simulink model "test_motor_model"  (Simulink 7.1)
settings: Solver=ode113  StartTime=0.0  StopTime=0.3  RelTol=1e-3
undefined symbols (not defined in the file or in its folder): Cog_sm, J_sm, Km_sm, L_sm, P0_sm, R_sm, Sm_sm
settings Model: Creator=dep06435  LastModifiedBy=dep06435  ExtModeTrigMode=oneshot  ExtModeArmWhenConnect=off
settings DataIOCC: LimitDataPoints=off  SaveOutput=off  SaveTime=off
settings OptimizationCC: BlockReduction=off  BooleanDataType=off
settings DebuggingCC: SaveWithParameterizedLinksMsg=none  SignalResolutionControl=TryResolveAllWithWarning  SolverPrmCheckMsg=none  MultiTaskDSMMsg=warning  MultiTaskCondExecSysMsg=none  StrictBusMsg=None
settings HardwareCC: TargetUnknown=on
settings RTWCC: IncludeERTFirstTime=on
settings STFCustomTargetCC: ModelReferenceCompliant=off  SystemTargetFile=grt.tlc

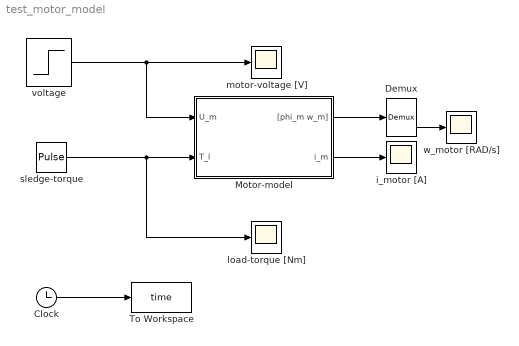
== system test_motor_model ==
  Clock : Clock
      settings: Decimation=10
  Demux : Demux  Outputs=2
  Motor-model : Subsystem  mask(Motor-model 1 VVR-41-AH-98004){km=Km_sm, Rm=R_sm, Jm=J_sm, Lm=L_sm, Sm=Sm_sm, Fc=Cog_sm, phim0=P0_sm}
      mask prompts: km "Motor-constant km [Nm/A]"; Rm "Motor-resistance R [ohm]"; Jm "Motor-inertia [kgm2]"; Lm "Motor-induction Lm [Vs/A]"; Sm "Stribeck minimal damping Sm [Nms/rad]"; Fc "Cogging-elements Fc [Nm]"; phim0 "Initial motor-position [rad]"
      mask help:
      | 2nd-order motor-model with non-linear Stribeck-damping
      | and cogging. State-vector "m" contains:
      |
      |       - motor-angle, -speed and -acceleration,
      |       - motor-current,
      |       - emk-voltage,
      |       - cogging-torque,
      |       - Stribeck-torque.
      |
      |   m = [phi_m  w_m  acc_m  i_m  U_emk
      |                                       T_cog  T_Stribeck]
  To Workspace : ToWorkspace  VariableName=time  SampleTime=-1  SaveFormat=Array
  i_motor [A] : Scope
      settings: TimeRange=0.5  YMin=0  YMax=0.225
  load-torque [Nm] : Scope
      settings: TimeRange=0.5  YMin=-1  YMax=1
  motor-voltage [V] : Scope
      settings: TimeRange=0.5  YMin=0  YMax=4
  sledge-torque : DiscretePulseGenerator  PulseType=Time based  Amplitude=0  Period=1  PulseWidth=50  PhaseDelay=0.00
  voltage : Step  Time=0.2  Before=4  After=-4  SampleTime=0
  w_motor [RAD/s] : Scope
      settings: TimeRange=0.5  YMin=-100  YMax=1300
  wires:
  voltage/1 -> motor-voltage [V]/1, Motor-model/1(U_m)
  Motor-model/2(i_m) -> i_motor [A]/1
  sledge-torque/1 -> Motor-model/2(T_l), load-torque [Nm]/1
  Motor-model/1("[phi_m w_m]") -> Demux/1
  Demux/2 -> w_motor [RAD/s]/1
  Clock/1 -> To Workspace/1

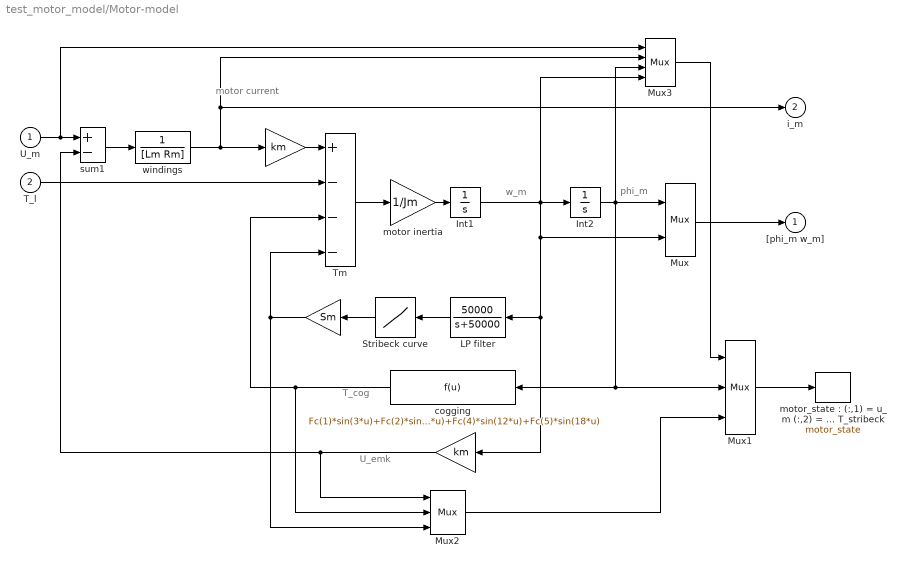
== system test_motor_model/Motor-model ==
  note: U_emk
  note: T_cog
  note: phi_m
  note: w_m
  note: motor
      | current
  U_m : Inport
  T_l : Inport  Port=2
  " " : Gain  Gain=km  SaturateOnIntegerOverflow=on  OutDataTypeStr=Inherit: Same as input  ParamDataTypeStr=Inherit: Same as input
  "      " : Gain  Orientation=left  Gain=km  SaturateOnIntegerOverflow=on  OutDataTypeStr=Inherit: Same as input  ParamDataTypeStr=Inherit: Same as input
  "     " : Gain  Orientation=left  Gain=Sm  SaturateOnIntegerOverflow=on  OutDataTypeStr=Inherit: Same as input  ParamDataTypeStr=Inherit: Same as input
  Int1 : Integrator
  Int2 : Integrator  InitialCondition=phim0
  LP filter : TransferFcn  Orientation=left  Numerator=[50000]  Denominator=[1 50000]
  Mux : Mux  Inputs=2
  Mux1 : Mux  Inputs=3
  Mux2 : Mux  Inputs=3
  Mux3 : Mux
  Stribeck curve : Lookup  Orientation=left  InputValues=[-2000,-200,-40,-30,-20,-10,-.01,0,.01,10,20,30,40,200,2000]  Table=[-1.859,-1,-1,-1.05,-1.15,-1.3,-1.5,0,1.5,1.3,1.15,1.05,1,1,1.859]  SaturateOnIntegerOverflow=on
  Tm : Sum  Inputs=+---  SaturateOnIntegerOverflow=on  InputSameDT=on  OutDataTypeStr=Inherit: Same as first input
  cogging : Fcn  Orientation=left  Expr=Fc(1)*sin(3*u)+Fc(2)*sin(6*u)+Fc(3)*sin(9*u)+Fc(4)*sin(12*u)+Fc(5)*sin(18*u)
  motor inertia : Gain  Gain=1/Jm  SaturateOnIntegerOverflow=on  OutDataTypeStr=Inherit: Same as input  ParamDataTypeStr=Inherit: Same as input
  "motor_state : (:,1) = u_m (:,2) = i_m (:,3) = phi_m (:,4) = w_m (:,5) = U_emk (:,6) = T_cog (:,7) = T_stribeck" : ToWorkspace  VariableName=motor_state  SampleTime=-1  SaveFormat=Array
  sum1 : Sum  Inputs=+-  SaturateOnIntegerOverflow=on  InputSameDT=on  OutDataTypeStr=Inherit: Same as first input
  windings : TransferFcn  Denominator=[Lm Rm]
  "[phi_m w_m]" : Outport
  i_m : Outport  Port=2
  wires:
  T_l/1 -> Tm/2
  sum1/1 -> windings/1
  windings/1 -> " "/1, i_m/1, Mux3/2
  " "/1 -> Tm/1
  Mux2/1 -> Mux1/3
  Int1/1 -> Mux/2, LP filter/1, "      "/1, Int2/1, Mux3/4
  Stribeck curve/1 -> "     "/1
  LP filter/1 -> Stribeck curve/1
  Int2/1 -> Mux/1, cogging/1, Mux1/2, Mux3/3
  Mux1/1 -> "motor_state : (:,1) = u_m (:,2) = i_m (:,3) = phi_m (:,4) = w_m (:,5) = U_emk (:,6) = T_cog (:,7) = T_stribeck"/1
  motor inertia/1 -> Int1/1
  U_m/1 -> sum1/1, Mux3/1
  Mux/1 -> "[phi_m w_m]"/1
  Mux3/1 -> Mux1/1
  "      "/1 -> sum1/2, Mux2/1
  cogging/1 -> Tm/3, Mux2/2
  "     "/1 -> Tm/4, Mux2/3
  Tm/1 -> motor inertia/1
